simulink model "problem4"  (R2020b)
settings: Solver=VariableStepAuto  StartTime=0.0  StopTime=10.0  RelTol=1e-3
libraries: dspsrcs4 x1
settings Model: Creator=admin  LastModifiedBy=admin

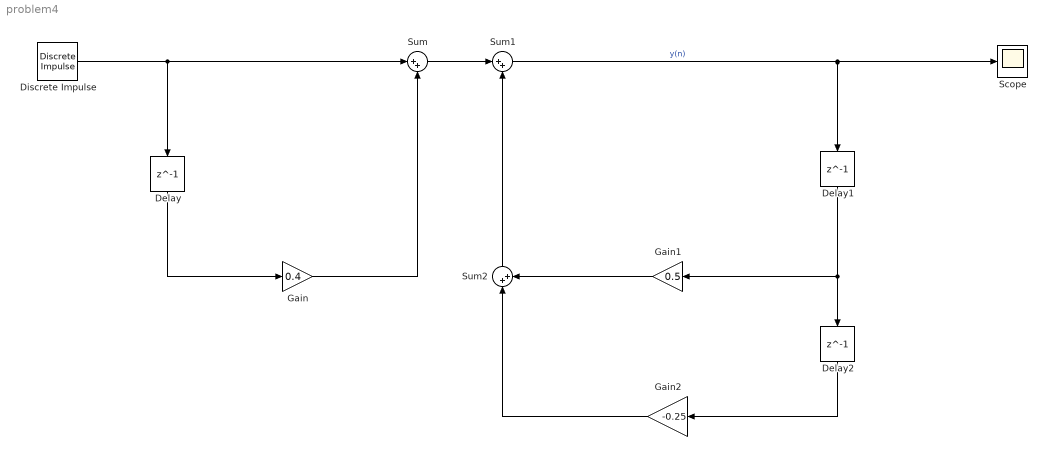
== system problem4 ==
  Delay : Delay  DelayLength=1  InitialCondition=0
  Delay1 : Delay  DelayLength=1  InitialCondition=0
  Delay2 : Delay  DelayLength=1  InitialCondition=0
  Discrete Impulse : dspsrcs4/Discrete  Impulse  Delay=0  SampleTime=1  FrameSample=1  OutputFrames=off  dataType=double  isSigned=on  wordLen=16  udDataType=sfix(16)  fracBitsMode=Best precision  numFracBits=15  OutDataTypeStr=double  LastOutDataTypeStr=double
  Gain : Gain  Gain=0.4
  Gain1 : Gain  Gain=0.5
  Gain2 : Gain  Gain=-0.25
  Scope : Scope
  Sum : Sum  Inputs=|++
  Sum1 : Sum  Inputs=|++
  Sum2 : Sum  Inputs=|++
  wires:
  Gain2/1 -> Sum2/1
  Gain1/1 -> Sum2/2
  Delay1/1 -> Delay2/1, Gain1/1
  Sum2/1 -> Sum1/2
  Sum1/1 -> Delay1/1, Scope/1  "y(n)"
  Delay2/1 -> Gain2/1
  Sum/1 -> Sum1/1
  Gain/1 -> Sum/2
  Delay/1 -> Gain/1
  Discrete Impulse/1 -> Delay/1, Sum/1
